simulink model "heatex_demo"  (Simulink 6.0)
settings: Solver=ode4  StartTime=0.0  StopTime=250  FixedStep=2  RelTol=1e-3
PreLoadFcn:
  | load heatex_demo
values from neighbouring files (symbols this model uses):
  Kf = -3    [pendulum_demo.mat]
  Ki = 0    [pendulum_demo.mat]    (also in servo_demo.mat)
  Kp = 4.81125224325    [pendulum_demo.mat]
  tau = 0.150156850627    [servo_demo.mat]
undefined symbols (not defined in the file or in its folder): DDelay
libraries: srolib x1
settings Model: Creator=pascal  LastModifiedBy=pascal
settings DataIOCC: SaveOutput=off  SaveTime=off  SignalLoggingName=logsOut
settings OptimizationCC: BlockReduction=off  BooleanDataType=off
settings DebuggingCC: CheckExecutionContextPreStartOutputMsg=on  CheckExecutionContextRuntimeOutputMsg=on  SolverPrmCheckMsg=none
settings HardwareCC: TargetUnknown=on
settings ModelReferenceCC: UpdateModelReferenceTargets=IfOutOfDate
settings GRTTargetCC: ModelReferenceCompliant=off
settings SFSimCC: SFSimApplyToAllLibs=on  SFSimBuildMode=Incremental

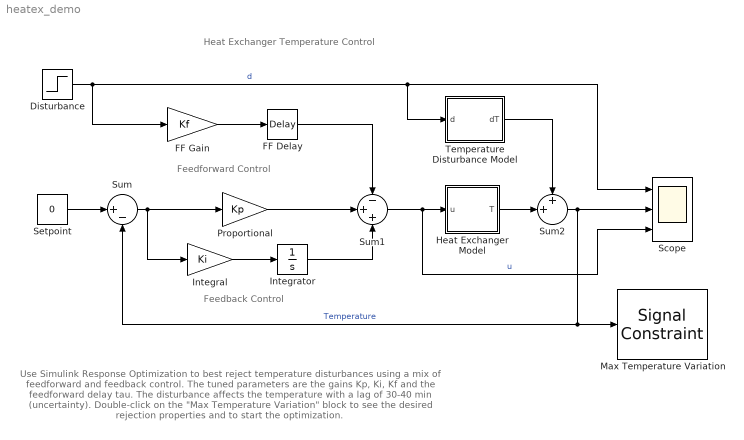
== system heatex_demo ==
  note: Feedback Control
  note: Feedforward Control
  note: Heat Exchanger Temperature Control
  note: Use Simulink Response Optimization to best reject temperature
      | disturbances using a mix of feedforward and feedback control.
      |
      | The tuned parameters are the gains Kp, Ki, Kf and the feedforward delay tau.
      | The disturbance affects the temperature with a lag of 30-40 min (uncertainty).
      |
      | Double-click on the "Max Temperature Variation" block to see the
      | desired rejection properties and to start the optimization.
  Disturbance : Step  Time=20  After=-1  SampleTime=0
  FF Delay : TransportDelay  DelayTime=tau
      settings: CloseFcn=disp('hello')
  FF Gain : Gain  Gain=Kf  SaturateOnIntegerOverflow=on
      settings: CloseFcn=disp('hello')
  Heat Exchanger Model : Subsystem  PropExecContextAcrossSSBoundary=on
  Integral : Gain  Gain=Ki  SaturateOnIntegerOverflow=on
  Integrator : Integrator
  Max Temperature Variation : srolib/Signal Constraint  DialogPosition=[0.046875 0.305833333333333 0.345625 0.245]  SaveIn=workspace  SaveAs=heatex_optim  LogID=SRO_DataLog_1  Ylim=[-0.6 0.6]
  Proportional : Gain  Gain=Kp  SaturateOnIntegerOverflow=on
  Scope : Scope  NumInputPorts=3
      settings: YMin=-1~-1~-1  YMax=1~1~1
  Setpoint : Constant  Value=0
  Sum : Sum  Inputs=|+-  SaturateOnIntegerOverflow=on  InputSameDT=on
  Sum1 : Sum  Inputs=-++  SaturateOnIntegerOverflow=on  InputSameDT=on
  Sum2 : Sum  Inputs=++|  SaturateOnIntegerOverflow=on  InputSameDT=on
  Temperature Disturbance Model : Subsystem  PropExecContextAcrossSSBoundary=on
  wires:
  Setpoint/1 -> Sum/1
  Sum/1 -> Proportional/1, Integral/1
  Sum1/1 -> Heat Exchanger Model/1(u), Scope/3  "u"
  Sum2/1 -> Scope/2, Sum/2, Max Temperature Variation/1  "Temperature"
  Disturbance/1 -> Temperature Disturbance Model/1(d), Scope/1, FF Gain/1  "d"
  Heat Exchanger Model/1(T) -> Sum2/2
  Temperature Disturbance Model/1(dT) -> Sum2/1
  Integral/1 -> Integrator/1
  Proportional/1 -> Sum1/2
  Integrator/1 -> Sum1/3
  FF Gain/1 -> FF Delay/1
  FF Delay/1 -> Sum1/1

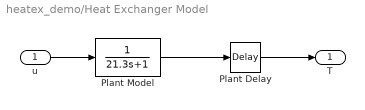
== system heatex_demo/Heat Exchanger Model ==
  u : Inport  LatchInput=off
  Plant Delay : TransportDelay  DelayTime=15
  Plant Model : TransferFcn  Denominator=[21.3 1]
  T : Outport
  wires:
  u/1 -> Plant Model/1
  Plant Model/1 -> Plant Delay/1
  Plant Delay/1 -> T/1

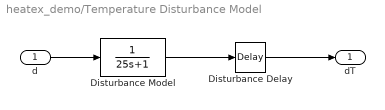
== system heatex_demo/Temperature Disturbance Model ==
  d : Inport  LatchInput=off
  Disturbance Delay : TransportDelay  DelayTime=DDelay
  Disturbance Model : TransferFcn  Denominator=[25 1]
  dT : Outport
  wires:
  Disturbance Delay/1 -> dT/1
  d/1 -> Disturbance Model/1
  Disturbance Model/1 -> Disturbance Delay/1
